simulink model "cruisecontrol"  (R2024a)
settings: Solver=FixedStepAuto  StartTime=0.0  StopTime=50  FixedStep=0.1  MaxStep=0.1  MinStep=0.1  RelTol=1e-3
model workspace (MAT data in the model file):
  b = 50
  m = 1000
  u = 500
settings Model: Creator=Jihoon  LastModifiedBy=Jihoon
settings SolverCC: InitialStep=0.1

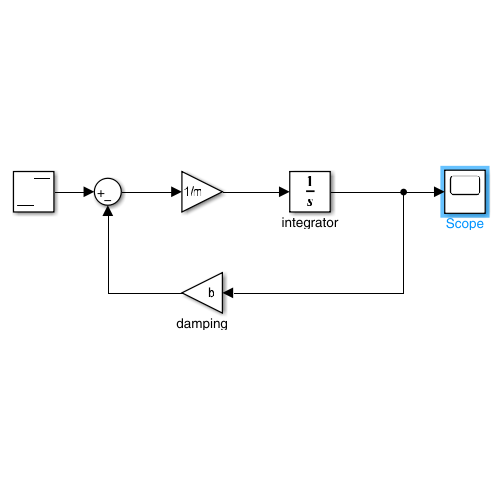
[thumbnail: Simulink's stored preview of the top-level diagram]
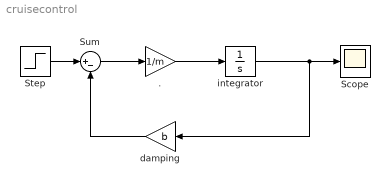
== system cruisecontrol ==
  . : Gain  Gain=1/m
  Scope : Scope
  Step : Step  Time=0  After=u  SampleTime=0
  Sum : Sum  Inputs=|+-
  damping : Gain  Gain=b
  integrator : Integrator
  wires:
  ./1 -> integrator/1
  Sum/1 -> ./1
  integrator/1 -> Scope/1, damping/1
  damping/1 -> Sum/2
  Step/1 -> Sum/1
